simulink model "user_defined_modules"  (R2022a)
settings: Solver=VariableStepAuto  StartTime=0.0  StopTime=10.0  RelTol=1e-3
settings Model: Creator=Home computer  LastModifiedBy=Home computer

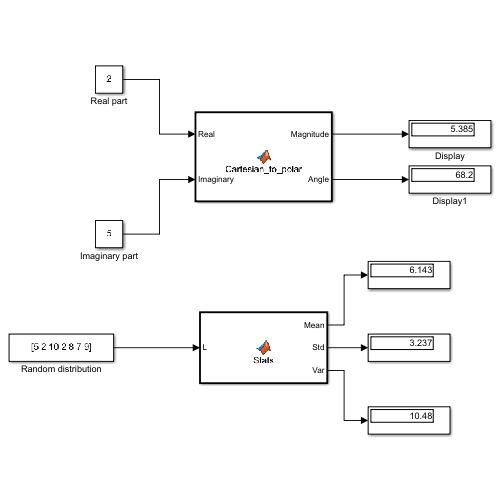
[thumbnail: Simulink's stored preview of the top-level diagram]
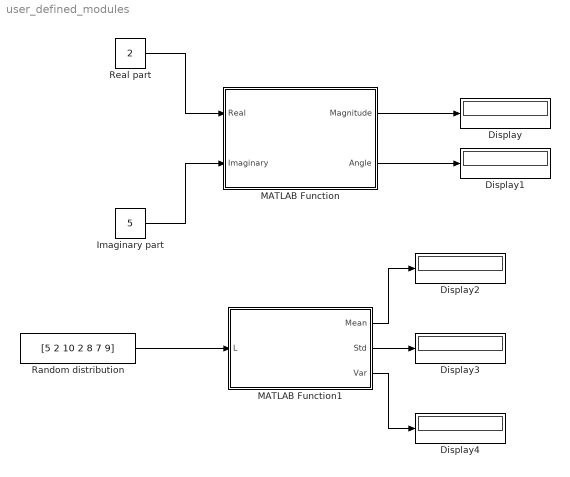
== system user_defined_modules ==
  Display{,1..4} (5 alike) : Display
  Imaginary part : Constant  Value=5
  MATLAB Function : MATLAB Function  TreatAsAtomicUnit=on
  MATLAB Function1 : MATLAB Function  TreatAsAtomicUnit=on
  Random distribution : Constant  Value=[5 2 10 2 8 7 9]
  Real part : Constant  Value=2
  wires:
  Real part/1 -> MATLAB Function/1(Real)
  Imaginary part/1 -> MATLAB Function/2(Imaginary)
  MATLAB Function/1(Magnitude) -> Display/1
  MATLAB Function/2(Angle) -> Display1/1
  MATLAB Function1/1(Mean) -> Display2/1
  MATLAB Function1/2(Std) -> Display3/1
  MATLAB Function1/3(Var) -> Display4/1
  Random distribution/1 -> MATLAB Function1/1(L)

== matlab function user_defined_modules/MATLAB Function ==
  data: Real input; Magnitude output; Imaginary input; Angle output
function [Magnitude, Angle] = Cartesian_to_polar(Real, Imaginary)
Magnitude = sqrt(Real^2 + Imaginary^2);
Angle = atan(Imaginary/Real) * (180/pi);

== matlab function user_defined_modules/MATLAB Function1 ==
  data: L input; Mean output; Std output; Var output
function [Mean, Std, Var] = Stats(L)
Mean = mean(L);
Std = std(L);
Var = var(L);
